simulink model "main-model"  (R2023a)
settings: Solver=FixedStepAuto  StartTime=0.0  StopTime=2.4  FixedStep=0.0001  RelTol=1e-3  AbsTol=1e-3
InitFcn:
  | addpath(fullfile(matlabroot,'toolbox/physmod/sm/sli/m'))
model workspace (MAT data in the model file):
  battery_cap = 0
  contingency_duration = 0.2
  contingency_time = 1.5
  final_demand = 1
  inertia_const = 0
  init_torque = 1.08
  response_time = 0.025
  solar_cap = 1
  solar_maxq = inf
  trans_time_const = 0
  transmission_lim = 1000
undefined symbols (not defined in the file or in its folder): ee
libraries: ee_lib x51, nesl_utility x34, fl_lib x30, eeTransforms x6, slpidlib x6, eeGeneralControl x6, eeSmAC1C x3, simulink x3, spsThreePhaseSineGeneratorLib x3, spsPLL3phLib x3
(part 3 of 3)

== system main-model/Bus 2/Solar Panel/Power Control ==
  Freq (Hz) : Inport
  Q (W) : Inport  Port=2
  Constant : Constant  Value=0
  Discrete PID Controller : slpidlib/PID Controller  Controller=PI  Form=Parallel  TimeDomain=Discrete-time  UseExternalTs=off  SampleTime=-1  IntegratorMethod=Forward Euler  FilterMethod=Forward Euler  ControllerParametersSource=internal  P=20  I=50  UseKiTs=off  D=0  N=100  UseFilter=on  TunerSelectOption=Transfer Function Based (PID Tuner App)  InitialConditionSource=internal  InitialConditionForIntegrator=0  InitialConditionForFilter=0  DifferentiatorICPrevScaledInput=0  ExternalReset=none  TrackingMode=off  Kt=1  LimitOutput=on  SatLimitsSource=internal  UpperSaturationLimit=solar_maxq  LowerSaturationLimit=-solar_maxq  LinearizeAsGain=off  AntiWindupMode=clamping  Kb=1  LimitIntegrator=off  UpperIntegratorSaturationLimit=inf  LowerIntegratorSaturationLimit=-inf  POutMin=[]  POutMax=[]  IOutMin=[]  IOutMax=[]  DOutMin=[]  DOutMax=[]  NOutMin=[]  NOutMax=[]  SumOutMin=[]  SumOutMax=[]  SaturationOutMin=[]  SaturationOutMax=[]  PParamMin=[]  PParamMax=[]  IParamMin=[]  IParamMax=[]  DParamMin=[]  DParamMax=[]  NParamMin=[]  NParamMax=[]  KbParamMin=[]  KbParamMax=[]  KtParamMin=[]  KtParamMax=[]  KbOutMin=[]  KbOutMax=[]  KtOutMin=[]  KtOutMax=[]  IntegratorOutMin=[]  IntegratorOutMax=[]  FilterOutMin=[]  FilterOutMax=[]  SumI1OutMin=[]  SumI1OutMax=[]  SumI2OutMin=[]  SumI2OutMax=[]  SumI3OutMin=[]  SumI3OutMax=[]  SumI4OutMin=[]  SumI4OutMax=[]  SumDOutMin=[]  SumDOutMax=[]  DifferentiatorOutMin=[]  DifferentiatorOutMax=[]  FilterDiffOutCoefMin=[]  FilterDiffOutCoefMax=[]  ReciprocalOutMin=[]  ReciprocalOutMax=[]  SumDenOutMin=[]  SumDenOutMax=[]  SumNumOutMin=[]  SumNumOutMax=[]  DivideOutMin=[]  DivideOutMax=[]  UdiffTsProdOutMin=[]  UdiffTsProdOutMax=[]  NTsProdOutMin=[]  NTsProdOutMax=[]  UintegralTsProdOutMin=[]  UintegralTsProdOutMax=[]  UngainTsProdOutMin=[]  UngainTsProdOutMax=[]  ClampingZeroOutDataTypeStr=Inherit: Inherit via back propagation  ClampingZeroOutMin=[]  ClampingZeroOutMax=[]  FilterDenConstantOutDataTypeStr=Inherit: Inherit via back propagation  FilterDenConstantOutMin=[]  FilterDenConstantOutMax=[]  PCopyOutDataTypeStr=Inherit: Inherit via back propagation  PCopyOutMin=[]  PCopyOutMax=[]  NCopyOutDataTypeStr=Inherit: Inherit via back propagation  NCopyOutMin=[]  NCopyOutMax=[]  IntegratorContinuousStateAttributes=''  IntegratorStateMustResolveToSignalObject=off  IntegratorRTWStateStorageClass=Auto  FilterContinuousStateAttributes=''  FilterStateMustResolveToSignalObject=off  FilterRTWStateStorageClass=Auto  ParallelPVariant=InternalParameters  IdealPVariant=Disabled  IVariant=InternalParameters  DVariant=Disabled  IntegratorVariant=Discrete  SatVariant=Enabled  AWVariant=DiscClampingParallel  PCopyVariant=Disabled  TRVariant=Disabled  FdbkBlocksVariant=Forward  IdealPFdbkVariant=Disabled  SatFdbkVariant=Disabled  DerivativeFilterVariant=Disabled  NVariant=Disabled  NCopyVariant=Disabled_SignalSpec  FilterICVariant=Disabled  IntegratorICVariant=InternalICs  ExternalResetVariant=Disabled  TRSumVariant=Passthrough  SumFdbkVariant=Disabled  SumVariant=Sum_PI  TsampFilterVariant=InternalTs  TsampNgainVariant=Passthrough  TsampIntegralVariant=Disabled_SignalSpec  ExternalSaturationOutDataTypeStr=Inherit: Same as second input
      settings: LibrarySourceBlock=simulink/Discrete/Discrete PID Controller
  Discrete PID Controller1 : slpidlib/PID Controller  Controller=PI  Form=Parallel  TimeDomain=Discrete-time  UseExternalTs=off  SampleTime=-1  IntegratorMethod=Forward Euler  FilterMethod=Forward Euler  ControllerParametersSource=internal  P=20  I=40  UseKiTs=off  D=0  N=100  UseFilter=off  TunerSelectOption=Transfer Function Based (PID Tuner App)  InitialConditionSource=internal  InitialConditionForIntegrator=0  InitialConditionForFilter=0  DifferentiatorICPrevScaledInput=0  ExternalReset=none  TrackingMode=off  Kt=1  LimitOutput=on  SatLimitsSource=internal  UpperSaturationLimit=inf  LowerSaturationLimit=1/solar_cap-1  LinearizeAsGain=off  AntiWindupMode=clamping  Kb=1  LimitIntegrator=off  UpperIntegratorSaturationLimit=inf  LowerIntegratorSaturationLimit=-inf  POutMin=[]  POutMax=[]  IOutMin=[]  IOutMax=[]  DOutMin=[]  DOutMax=[]  NOutMin=[]  NOutMax=[]  SumOutMin=[]  SumOutMax=[]  SaturationOutMin=[]  SaturationOutMax=[]  PParamMin=[]  PParamMax=[]  IParamMin=[]  IParamMax=[]  DParamMin=[]  DParamMax=[]  NParamMin=[]  NParamMax=[]  KbParamMin=[]  KbParamMax=[]  KtParamMin=[]  KtParamMax=[]  KbOutMin=[]  KbOutMax=[]  KtOutMin=[]  KtOutMax=[]  IntegratorOutMin=[]  IntegratorOutMax=[]  FilterOutMin=[]  FilterOutMax=[]  SumI1OutMin=[]  SumI1OutMax=[]  SumI2OutMin=[]  SumI2OutMax=[]  SumI3OutMin=[]  SumI3OutMax=[]  SumI4OutMin=[]  SumI4OutMax=[]  SumDOutMin=[]  SumDOutMax=[]  DifferentiatorOutMin=[]  DifferentiatorOutMax=[]  FilterDiffOutCoefMin=[]  FilterDiffOutCoefMax=[]  ReciprocalOutMin=[]  ReciprocalOutMax=[]  SumDenOutMin=[]  SumDenOutMax=[]  SumNumOutMin=[]  SumNumOutMax=[]  DivideOutMin=[]  DivideOutMax=[]  UdiffTsProdOutMin=[]  UdiffTsProdOutMax=[]  NTsProdOutMin=[]  NTsProdOutMax=[]  UintegralTsProdOutMin=[]  UintegralTsProdOutMax=[]  UngainTsProdOutMin=[]  UngainTsProdOutMax=[]  ClampingZeroOutDataTypeStr=Inherit: Inherit via back propagation  ClampingZeroOutMin=[]  ClampingZeroOutMax=[]  FilterDenConstantOutDataTypeStr=Inherit: Inherit via back propagation  FilterDenConstantOutMin=[]  FilterDenConstantOutMax=[]  PCopyOutDataTypeStr=Inherit: Inherit via back propagation  PCopyOutMin=[]  PCopyOutMax=[]  NCopyOutDataTypeStr=Inherit: Inherit via back propagation  NCopyOutMin=[]  NCopyOutMax=[]  IntegratorContinuousStateAttributes=''  IntegratorStateMustResolveToSignalObject=off  IntegratorRTWStateStorageClass=Auto  FilterContinuousStateAttributes=''  FilterStateMustResolveToSignalObject=off  FilterRTWStateStorageClass=Auto  ParallelPVariant=InternalParameters  IdealPVariant=Disabled  IVariant=InternalParameters  DVariant=Disabled  IntegratorVariant=Discrete  SatVariant=Enabled  AWVariant=DiscClampingParallel  PCopyVariant=Disabled  TRVariant=Disabled  FdbkBlocksVariant=Forward  IdealPFdbkVariant=Disabled  SatFdbkVariant=Disabled  DerivativeFilterVariant=Disabled  NVariant=Disabled  NCopyVariant=Disabled_SignalSpec  FilterICVariant=Disabled  IntegratorICVariant=InternalICs  ExternalResetVariant=Disabled  TRSumVariant=Passthrough  SumFdbkVariant=Disabled  SumVariant=Sum_PI  TsampFilterVariant=InternalTs  TsampNgainVariant=Passthrough  TsampIntegralVariant=Disabled_SignalSpec  ExternalSaturationOutDataTypeStr=Inherit: Same as second input
      settings: LibrarySourceBlock=simulink/Discrete/Discrete PID Controller
  Load Set : Constant  Value=1/solar_cap
  Low-Pass Filter (Discrete or Continuous) : eeGeneralControl/Low-Pass Filter (Discrete or Continuous)  K=1  T=0.1  B=inf  A=-inf  init_option=Specify as parameter  x0=0  Ts=-1
  Rate Limiter : RateLimiter  RisingSlewLimit=1.5  FallingSlewLimit=-1.5  SampleTimeMode=inherited  InitialCondition=1/solar_cap
  Ref Freq : Constant
  SI to pu : Gain  Gain=1/60
  SI to pu1 : Gain  Gain=1/(solar_cap*0.8*load*10^6)
  Sum : Sum  Inputs=-+|
  Sum1 : Sum  Inputs=+-|
  Sum2 : Sum  Inputs=|-+
  Pset (pu) : Outport
  Qset (pu) : Outport  Port=2
  wires:
  SI to pu1/1 -> Low-Pass Filter (Discrete or Continuous)/1
  Constant/1 -> Sum2/2
  Low-Pass Filter (Discrete or Continuous)/1 -> Sum2/1
  Discrete PID Controller/1 -> Qset (pu)/1
  Q (W)/1 -> SI to pu1/1
  Rate Limiter/1 -> Pset (pu)/1
  Sum1/1 -> Rate Limiter/1
  Discrete PID Controller1/1 -> Sum1/2
  Sum/1 -> Discrete PID Controller1/1
  Load Set/1 -> Sum1/1
  Ref Freq/1 -> Sum/1
  SI to pu/1 -> Sum/2
  Freq (Hz)/1 -> SI to pu/1
  Sum2/1 -> Discrete PID Controller/1

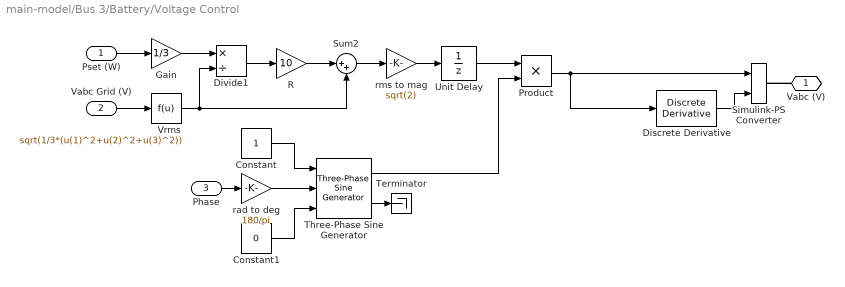
== system main-model/Bus 3/Battery/Voltage Control ==
  Pset (W) : Inport
  Vabc Grid (V) : Inport  Port=2
  Phase : Inport  Port=3
  Constant : Constant
  Constant1 : Constant  Value=0
  Discrete Derivative : simulink/Discrete/Discrete Derivative  gainval=1.0  ICPrevScaledInput=0.0  OutMin=[]  OutMax=[]  OutDataType=fixdt(1, 16)  OutScaling=2^-10  DoSatur=off
  Divide1 : Product  Inputs=*/
  Gain : Gain  Gain=1/3
  Product : Product
  R : Gain  Gain=10
  Simulink-PS Converter : nesl_utility/Simulink-PS Converter  PhysicalDomain=network_engine_domain  SubClassName=ps_input  LeftPortType=input  RightPortType=output  PseudoPeriodic=off  Frequencies=[]  NoiseDistribution=none  NoiseParameters=[]  Unit=V  AffineConversion=off  FilteringAndDerivatives=provide  SimscapeFilterOrder=1  InputFilterTimeConstant=1e-4  UdotUserProvided=1
  Sum2 : Sum  Inputs=|++
  Terminator : Terminator
  Three-Phase Sine Generator : spsThreePhaseSineGeneratorLib/Three-Phase Sine Generator  Ts=0
      settings: LibrarySourceBlock=|
      | sps_lib/Sources/Signal Generator Sources/Three-Phase
      | Sine Generator
  Unit Delay : UnitDelay  InitialCondition=350*sqrt(2)*10^3  SampleTime=-1  HasFrameUpgradeWarning=on
  Vrms : Fcn  Expr=sqrt(1/3*(u(1)^2+u(2)^2+u(3)^2))
  rad to deg : Gain  Gain=180/pi
  rms to mag : Gain  Gain=sqrt(2)
  Vabc (V) : PMIOPort  Side=Right
  wires:
  Discrete Derivative/1 -> Simulink-PS Converter/2
  Vabc Grid (V)/1 -> Vrms/1
  Pset (W)/1 -> Gain/1
  Divide1/1 -> R/1
  R/1 -> Sum2/1
  Gain/1 -> Divide1/1
  Sum2/1 -> rms to mag/1
  Vrms/1 -> Sum2/2, Divide1/2
  Phase/1 -> rad to deg/1
  Constant/1 -> Three-Phase Sine Generator/1
  Constant1/1 -> Three-Phase Sine Generator/3
  Three-Phase Sine Generator/2 -> Terminator/1
  Three-Phase Sine Generator/1 -> Product/2
  rad to deg/1 -> Three-Phase Sine Generator/2
  rms to mag/1 -> Unit Delay/1
  Product/1 -> Discrete Derivative/1, Simulink-PS Converter/1
  Unit Delay/1 -> Product/1
  connections:
  Vabc (V)/RConn1 -- Simulink-PS Converter/RConn1

== system main-model/Bus 3/Governor and Prime Mover/Governor ==
  pu_velocity : Inport
  1/T_G : Gain  Gain=1/T_G
  1/droop : Gain  Gain=1/(droop_percentage/100)
  Delta load setpoint : Sum  Inputs=+-|
  Delta speed : Sum  Inputs=-+|
  Integrator : Integrator  InitialCondition=pu_torque0
  Load_setpoint : Constant  Value=pu_load_reference_setpoint
  Saturation : Saturate  UpperLimit=max_torque  LowerLimit=0
  Speed_ref : Constant  Value=pu_speed_reference
  Subtract : Sum  Inputs=|+-
  delta_y : Outport  VectorParamsAs1DForOutWhenUnconnected=off
  wires:
  Speed_ref/1 -> Delta speed/1
  Delta speed/1 -> 1/droop/1
  Load_setpoint/1 -> Delta load setpoint/1
  pu_velocity/1 -> Delta speed/2
  1/droop/1 -> Delta load setpoint/2
  1/T_G/1 -> Integrator/1
  Integrator/1 -> delta_y/1, Subtract/2
  Subtract/1 -> 1/T_G/1
  Delta load setpoint/1 -> Saturation/1
  Saturation/1 -> Subtract/1

== system main-model/Bus 3/Governor and Prime Mover/Non-reheat turbine ==
  delta_y : Inport
  1/T_CH : Gain  Gain=1/T_CH
  Integrator : Integrator  InitialCondition=pu_torque0  UpperSaturationLimit=max_torque
  Sum : Sum  Inputs=|+-
  torque : Outport  VectorParamsAs1DForOutWhenUnconnected=off
  wires:
  delta_y/1 -> Sum/1
  Sum/1 -> 1/T_CH/1
  1/T_CH/1 -> Integrator/1
  Integrator/1 -> Sum/2, torque/1

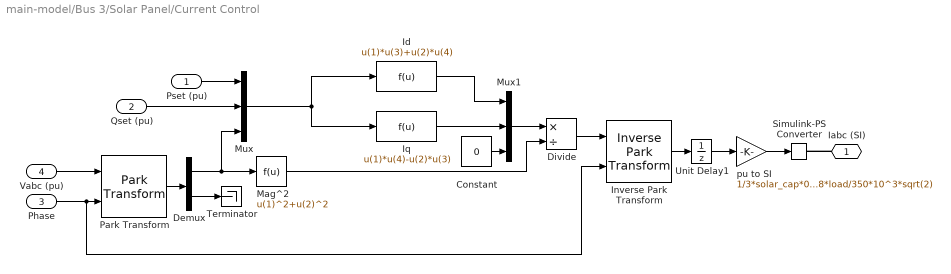
== system main-model/Bus 3/Solar Panel/Current Control ==
  Pset (pu) : Inport
  Qset (pu) : Inport  Port=2
  Phase : Inport  Port=3
  Vabc (pu) : Inport  Port=4
  Constant : Constant  Value=0
  Demux : Demux  Outputs=[2 1]
  Divide : Product  Inputs=*/
  Id : Fcn  Expr=u(1)*u(3)+u(2)*u(4)
  Inverse Park Transform : eeTransforms/Inverse Park Transform  AxisAlignment=Q-axis  PowerInvariant=off
      settings: LibrarySourceBlock=|
      | ee_sl_lib/Mathematical
      | Transforms/Inverse
      | Park Transform
  Iq : Fcn  Expr=u(1)*u(4)-u(2)*u(3)
  Mag^2 : Fcn  Expr=u(1)^2+u(2)^2
  Mux : Mux  Inputs=3
  Mux1 : Mux  Inputs=3
  Park Transform : eeTransforms/Park Transform  AxisAlignment=Q-axis  PowerInvariant=off
      settings: LibrarySourceBlock=|
      | ee_sl_lib/Mathematical
      | Transforms/Park Transform
  Simulink-PS Converter : nesl_utility/Simulink-PS Converter  PhysicalDomain=network_engine_domain  SubClassName=ps_input  LeftPortType=input  RightPortType=output  PseudoPeriodic=off  Frequencies=[]  NoiseDistribution=none  NoiseParameters=[]  Unit=A  AffineConversion=off  FilteringAndDerivatives=filter  SimscapeFilterOrder=1  InputFilterTimeConstant=1e-4  UdotUserProvided=0
  Terminator : Terminator
  Unit Delay1 : UnitDelay  InitialCondition=1/solar_cap*[0 -sin(2*pi/3) sin(2*pi/3)]  SampleTime=-1  HasFrameUpgradeWarning=on
  pu to SI : Gain  Gain=1/3*solar_cap*0.8*load/350*10^3*sqrt(2)
  Iabc (SI) : PMIOPort  Side=Right
  wires:
  Park Transform/1 -> Demux/1
  Demux/2 -> Terminator/1
  Demux/1 -> Mux/3, Mag^2/1
  Mag^2/1 -> Divide/2
  pu to SI/1 -> Simulink-PS Converter/1
  Constant/1 -> Mux1/3
  Phase/1 -> Inverse Park Transform/2, Park Transform/2
  Vabc (pu)/1 -> Park Transform/1
  Id/1 -> Mux1/1
  Iq/1 -> Mux1/2
  Inverse Park Transform/1 -> Unit Delay1/1
  Unit Delay1/1 -> pu to SI/1
  Mux1/1 -> Divide/1
  Divide/1 -> Inverse Park Transform/1
  Pset (pu)/1 -> Mux/1
  Qset (pu)/1 -> Mux/2
  Mux/1 -> Id/1, Iq/1
  connections:
  Iabc (SI)/RConn1 -- Simulink-PS Converter/RConn1

== system main-model/Bus 3/Solar Panel/Power Control ==
  Freq (Hz) : Inport
  Q (W) : Inport  Port=2
  Constant : Constant  Value=0
  Discrete PID Controller : slpidlib/PID Controller  Controller=PI  Form=Parallel  TimeDomain=Discrete-time  UseExternalTs=off  SampleTime=-1  IntegratorMethod=Forward Euler  FilterMethod=Forward Euler  ControllerParametersSource=internal  P=20  I=50  UseKiTs=off  D=0  N=100  UseFilter=on  TunerSelectOption=Transfer Function Based (PID Tuner App)  InitialConditionSource=internal  InitialConditionForIntegrator=0  InitialConditionForFilter=0  DifferentiatorICPrevScaledInput=0  ExternalReset=none  TrackingMode=off  Kt=1  LimitOutput=on  SatLimitsSource=internal  UpperSaturationLimit=solar_maxq  LowerSaturationLimit=-solar_maxq  LinearizeAsGain=off  AntiWindupMode=clamping  Kb=1  LimitIntegrator=off  UpperIntegratorSaturationLimit=inf  LowerIntegratorSaturationLimit=-inf  POutMin=[]  POutMax=[]  IOutMin=[]  IOutMax=[]  DOutMin=[]  DOutMax=[]  NOutMin=[]  NOutMax=[]  SumOutMin=[]  SumOutMax=[]  SaturationOutMin=[]  SaturationOutMax=[]  PParamMin=[]  PParamMax=[]  IParamMin=[]  IParamMax=[]  DParamMin=[]  DParamMax=[]  NParamMin=[]  NParamMax=[]  KbParamMin=[]  KbParamMax=[]  KtParamMin=[]  KtParamMax=[]  KbOutMin=[]  KbOutMax=[]  KtOutMin=[]  KtOutMax=[]  IntegratorOutMin=[]  IntegratorOutMax=[]  FilterOutMin=[]  FilterOutMax=[]  SumI1OutMin=[]  SumI1OutMax=[]  SumI2OutMin=[]  SumI2OutMax=[]  SumI3OutMin=[]  SumI3OutMax=[]  SumI4OutMin=[]  SumI4OutMax=[]  SumDOutMin=[]  SumDOutMax=[]  DifferentiatorOutMin=[]  DifferentiatorOutMax=[]  FilterDiffOutCoefMin=[]  FilterDiffOutCoefMax=[]  ReciprocalOutMin=[]  ReciprocalOutMax=[]  SumDenOutMin=[]  SumDenOutMax=[]  SumNumOutMin=[]  SumNumOutMax=[]  DivideOutMin=[]  DivideOutMax=[]  UdiffTsProdOutMin=[]  UdiffTsProdOutMax=[]  NTsProdOutMin=[]  NTsProdOutMax=[]  UintegralTsProdOutMin=[]  UintegralTsProdOutMax=[]  UngainTsProdOutMin=[]  UngainTsProdOutMax=[]  ClampingZeroOutDataTypeStr=Inherit: Inherit via back propagation  ClampingZeroOutMin=[]  ClampingZeroOutMax=[]  FilterDenConstantOutDataTypeStr=Inherit: Inherit via back propagation  FilterDenConstantOutMin=[]  FilterDenConstantOutMax=[]  PCopyOutDataTypeStr=Inherit: Inherit via back propagation  PCopyOutMin=[]  PCopyOutMax=[]  NCopyOutDataTypeStr=Inherit: Inherit via back propagation  NCopyOutMin=[]  NCopyOutMax=[]  IntegratorContinuousStateAttributes=''  IntegratorStateMustResolveToSignalObject=off  IntegratorRTWStateStorageClass=Auto  FilterContinuousStateAttributes=''  FilterStateMustResolveToSignalObject=off  FilterRTWStateStorageClass=Auto  ParallelPVariant=InternalParameters  IdealPVariant=Disabled  IVariant=InternalParameters  DVariant=Disabled  IntegratorVariant=Discrete  SatVariant=Enabled  AWVariant=DiscClampingParallel  PCopyVariant=Disabled  TRVariant=Disabled  FdbkBlocksVariant=Forward  IdealPFdbkVariant=Disabled  SatFdbkVariant=Disabled  DerivativeFilterVariant=Disabled  NVariant=Disabled  NCopyVariant=Disabled_SignalSpec  FilterICVariant=Disabled  IntegratorICVariant=InternalICs  ExternalResetVariant=Disabled  TRSumVariant=Passthrough  SumFdbkVariant=Disabled  SumVariant=Sum_PI  TsampFilterVariant=InternalTs  TsampNgainVariant=Passthrough  TsampIntegralVariant=Disabled_SignalSpec  ExternalSaturationOutDataTypeStr=Inherit: Same as second input
      settings: LibrarySourceBlock=simulink/Discrete/Discrete PID Controller
  Discrete PID Controller1 : slpidlib/PID Controller  Controller=PI  Form=Parallel  TimeDomain=Discrete-time  UseExternalTs=off  SampleTime=-1  IntegratorMethod=Forward Euler  FilterMethod=Forward Euler  ControllerParametersSource=internal  P=20  I=40  UseKiTs=off  D=0  N=100  UseFilter=off  TunerSelectOption=Transfer Function Based (PID Tuner App)  InitialConditionSource=internal  InitialConditionForIntegrator=0  InitialConditionForFilter=0  DifferentiatorICPrevScaledInput=0  ExternalReset=none  TrackingMode=off  Kt=1  LimitOutput=on  SatLimitsSource=internal  UpperSaturationLimit=inf  LowerSaturationLimit=1/solar_cap-1  LinearizeAsGain=off  AntiWindupMode=clamping  Kb=1  LimitIntegrator=off  UpperIntegratorSaturationLimit=inf  LowerIntegratorSaturationLimit=-inf  POutMin=[]  POutMax=[]  IOutMin=[]  IOutMax=[]  DOutMin=[]  DOutMax=[]  NOutMin=[]  NOutMax=[]  SumOutMin=[]  SumOutMax=[]  SaturationOutMin=[]  SaturationOutMax=[]  PParamMin=[]  PParamMax=[]  IParamMin=[]  IParamMax=[]  DParamMin=[]  DParamMax=[]  NParamMin=[]  NParamMax=[]  KbParamMin=[]  KbParamMax=[]  KtParamMin=[]  KtParamMax=[]  KbOutMin=[]  KbOutMax=[]  KtOutMin=[]  KtOutMax=[]  IntegratorOutMin=[]  IntegratorOutMax=[]  FilterOutMin=[]  FilterOutMax=[]  SumI1OutMin=[]  SumI1OutMax=[]  SumI2OutMin=[]  SumI2OutMax=[]  SumI3OutMin=[]  SumI3OutMax=[]  SumI4OutMin=[]  SumI4OutMax=[]  SumDOutMin=[]  SumDOutMax=[]  DifferentiatorOutMin=[]  DifferentiatorOutMax=[]  FilterDiffOutCoefMin=[]  FilterDiffOutCoefMax=[]  ReciprocalOutMin=[]  ReciprocalOutMax=[]  SumDenOutMin=[]  SumDenOutMax=[]  SumNumOutMin=[]  SumNumOutMax=[]  DivideOutMin=[]  DivideOutMax=[]  UdiffTsProdOutMin=[]  UdiffTsProdOutMax=[]  NTsProdOutMin=[]  NTsProdOutMax=[]  UintegralTsProdOutMin=[]  UintegralTsProdOutMax=[]  UngainTsProdOutMin=[]  UngainTsProdOutMax=[]  ClampingZeroOutDataTypeStr=Inherit: Inherit via back propagation  ClampingZeroOutMin=[]  ClampingZeroOutMax=[]  FilterDenConstantOutDataTypeStr=Inherit: Inherit via back propagation  FilterDenConstantOutMin=[]  FilterDenConstantOutMax=[]  PCopyOutDataTypeStr=Inherit: Inherit via back propagation  PCopyOutMin=[]  PCopyOutMax=[]  NCopyOutDataTypeStr=Inherit: Inherit via back propagation  NCopyOutMin=[]  NCopyOutMax=[]  IntegratorContinuousStateAttributes=''  IntegratorStateMustResolveToSignalObject=off  IntegratorRTWStateStorageClass=Auto  FilterContinuousStateAttributes=''  FilterStateMustResolveToSignalObject=off  FilterRTWStateStorageClass=Auto  ParallelPVariant=InternalParameters  IdealPVariant=Disabled  IVariant=InternalParameters  DVariant=Disabled  IntegratorVariant=Discrete  SatVariant=Enabled  AWVariant=DiscClampingParallel  PCopyVariant=Disabled  TRVariant=Disabled  FdbkBlocksVariant=Forward  IdealPFdbkVariant=Disabled  SatFdbkVariant=Disabled  DerivativeFilterVariant=Disabled  NVariant=Disabled  NCopyVariant=Disabled_SignalSpec  FilterICVariant=Disabled  IntegratorICVariant=InternalICs  ExternalResetVariant=Disabled  TRSumVariant=Passthrough  SumFdbkVariant=Disabled  SumVariant=Sum_PI  TsampFilterVariant=InternalTs  TsampNgainVariant=Passthrough  TsampIntegralVariant=Disabled_SignalSpec  ExternalSaturationOutDataTypeStr=Inherit: Same as second input
      settings: LibrarySourceBlock=simulink/Discrete/Discrete PID Controller
  Load Set : Constant  Value=1/solar_cap
  Low-Pass Filter (Discrete or Continuous) : eeGeneralControl/Low-Pass Filter (Discrete or Continuous)  K=1  T=0.1  B=inf  A=-inf  init_option=Specify as parameter  x0=0  Ts=-1
  Rate Limiter : RateLimiter  RisingSlewLimit=1.5  FallingSlewLimit=-1.5  SampleTimeMode=inherited  InitialCondition=1/solar_cap
  Ref Freq : Constant
  SI to pu : Gain  Gain=1/60
  SI to pu1 : Gain  Gain=1/(solar_cap*0.8*load*10^6)
  Sum : Sum  Inputs=-+|
  Sum1 : Sum  Inputs=+-|
  Sum2 : Sum  Inputs=|-+
  Pset (pu) : Outport
  Qset (pu) : Outport  Port=2
  wires:
  Sum2/1 -> Discrete PID Controller/1
  Freq (Hz)/1 -> SI to pu/1
  SI to pu/1 -> Sum/2
  Ref Freq/1 -> Sum/1
  Load Set/1 -> Sum1/1
  Sum/1 -> Discrete PID Controller1/1
  Discrete PID Controller1/1 -> Sum1/2
  Sum1/1 -> Rate Limiter/1
  Rate Limiter/1 -> Pset (pu)/1
  Q (W)/1 -> SI to pu1/1
  Discrete PID Controller/1 -> Qset (pu)/1
  Low-Pass Filter (Discrete or Continuous)/1 -> Sum2/1
  Constant/1 -> Sum2/2
  SI to pu1/1 -> Low-Pass Filter (Discrete or Continuous)/1
